simulink model "four_bit_adder"  (R2017a)
settings: Solver=VariableStepAuto  StartTime=0.0  StopTime=10.0  RelTol=1e-3
settings Model: Creator=nailt  LastModifiedBy=nailt

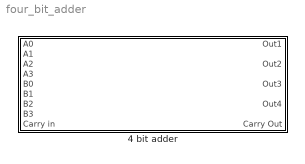
== system four_bit_adder ==
  4 bit adder : Subsystem

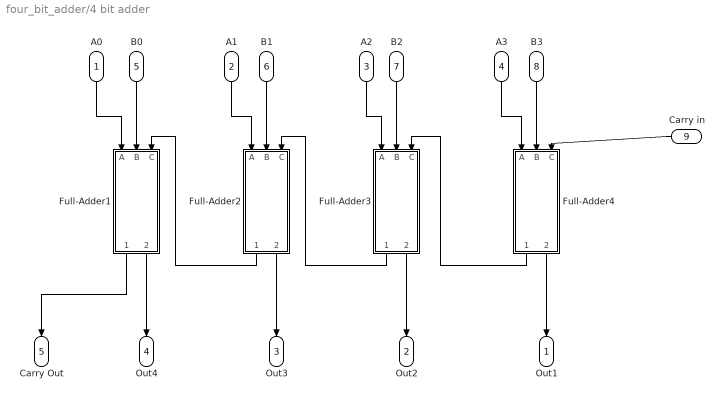
== system four_bit_adder/4 bit adder ==
  "A0 " : Inport
  "A1 " : Inport  Port=2
  A2 : Inport  Port=3
  A3 : Inport  Port=4
  B0 : Inport  Port=5
  B1 : Inport  Port=6
  B2 : Inport  Port=7
  B3 : Inport  Port=8
  Carry in : Inport  Port=9
  Full-Adder1 : Subsystem
  Full-Adder2 : Subsystem
  Full-Adder3 : Subsystem
  Full-Adder4 : Subsystem
  Out1 : Outport
  Out2 : Outport  Port=2
  Out3 : Outport  Port=3
  Out4 : Outport  Port=4
  Carry Out : Outport  Port=5
  wires:
  B3/1 -> Full-Adder4/2(B)
  B2/1 -> Full-Adder3/2(B)
  Full-Adder1/1(CARRY) -> Carry Out/1
  A3/1 -> Full-Adder4/1(A)
  "A1 "/1 -> Full-Adder2/1(A)
  Full-Adder2/1(CARRY) -> Full-Adder1/3(C)
  "A0 "/1 -> Full-Adder1/1(A)
  Full-Adder3/2(OUTPUT) -> Out2/1
  B1/1 -> Full-Adder2/2(B)
  Full-Adder4/2(OUTPUT) -> Out1/1
  Full-Adder2/2(OUTPUT) -> Out3/1
  Carry in/1 -> Full-Adder4/3(C)
  Full-Adder1/2(OUTPUT) -> Out4/1
  Full-Adder4/1(CARRY) -> Full-Adder3/3(C)
  A2/1 -> Full-Adder3/1(A)
  Full-Adder3/1(CARRY) -> Full-Adder2/3(C)
  B0/1 -> Full-Adder1/2(B)

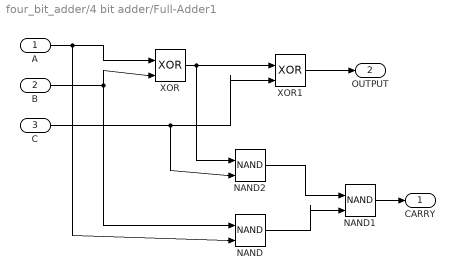
== system four_bit_adder/4 bit adder/Full-Adder1 ==
  A : Inport
  B : Inport  Port=2
  C : Inport  Port=3
  NAND : Logic  Operator=NAND  IconShape=distinctive  AllPortsSameDT=off  OutDataTypeStr=boolean
  NAND1 : Logic  Operator=NAND  IconShape=distinctive  AllPortsSameDT=off  OutDataTypeStr=boolean
  NAND2 : Logic  Operator=NAND  IconShape=distinctive  AllPortsSameDT=off  OutDataTypeStr=boolean
  XOR : Logic  Operator=XOR  IconShape=distinctive  AllPortsSameDT=off  OutDataTypeStr=boolean
  XOR1 : Logic  Operator=XOR  IconShape=distinctive  AllPortsSameDT=off  OutDataTypeStr=boolean
  CARRY : Outport
  OUTPUT : Outport  Port=2
  wires:
  C/1 -> NAND2/2, XOR1/2
  XOR1/1 -> OUTPUT/1
  A/1 -> NAND/2, XOR/1
  B/1 -> NAND/1, XOR/2
  NAND/1 -> NAND1/2
  NAND1/1 -> CARRY/1
  NAND2/1 -> NAND1/1
  XOR/1 -> NAND2/1, XOR1/1

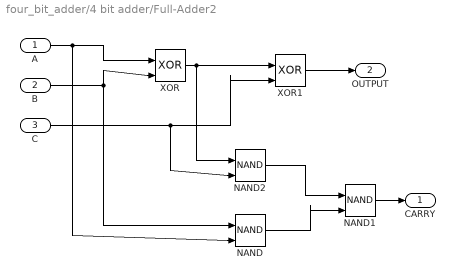
== system four_bit_adder/4 bit adder/Full-Adder2 ==
  A : Inport
  B : Inport  Port=2
  C : Inport  Port=3
  NAND : Logic  Operator=NAND  IconShape=distinctive  AllPortsSameDT=off  OutDataTypeStr=boolean
  NAND1 : Logic  Operator=NAND  IconShape=distinctive  AllPortsSameDT=off  OutDataTypeStr=boolean
  NAND2 : Logic  Operator=NAND  IconShape=distinctive  AllPortsSameDT=off  OutDataTypeStr=boolean
  XOR : Logic  Operator=XOR  IconShape=distinctive  AllPortsSameDT=off  OutDataTypeStr=boolean
  XOR1 : Logic  Operator=XOR  IconShape=distinctive  AllPortsSameDT=off  OutDataTypeStr=boolean
  CARRY : Outport
  OUTPUT : Outport  Port=2
  wires:
  C/1 -> NAND2/2, XOR1/2
  XOR1/1 -> OUTPUT/1
  A/1 -> NAND/2, XOR/1
  B/1 -> NAND/1, XOR/2
  NAND/1 -> NAND1/2
  NAND1/1 -> CARRY/1
  NAND2/1 -> NAND1/1
  XOR/1 -> NAND2/1, XOR1/1

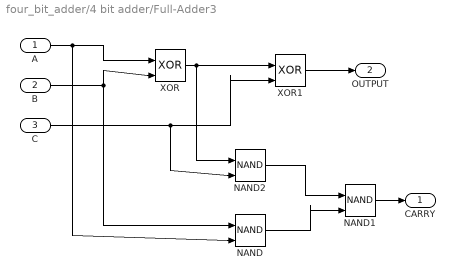
== system four_bit_adder/4 bit adder/Full-Adder3 ==
  A : Inport
  B : Inport  Port=2
  C : Inport  Port=3
  NAND : Logic  Operator=NAND  IconShape=distinctive  AllPortsSameDT=off  OutDataTypeStr=boolean
  NAND1 : Logic  Operator=NAND  IconShape=distinctive  AllPortsSameDT=off  OutDataTypeStr=boolean
  NAND2 : Logic  Operator=NAND  IconShape=distinctive  AllPortsSameDT=off  OutDataTypeStr=boolean
  XOR : Logic  Operator=XOR  IconShape=distinctive  AllPortsSameDT=off  OutDataTypeStr=boolean
  XOR1 : Logic  Operator=XOR  IconShape=distinctive  AllPortsSameDT=off  OutDataTypeStr=boolean
  CARRY : Outport
  OUTPUT : Outport  Port=2
  wires:
  C/1 -> NAND2/2, XOR1/2
  XOR1/1 -> OUTPUT/1
  A/1 -> NAND/2, XOR/1
  B/1 -> NAND/1, XOR/2
  NAND/1 -> NAND1/2
  NAND1/1 -> CARRY/1
  NAND2/1 -> NAND1/1
  XOR/1 -> NAND2/1, XOR1/1

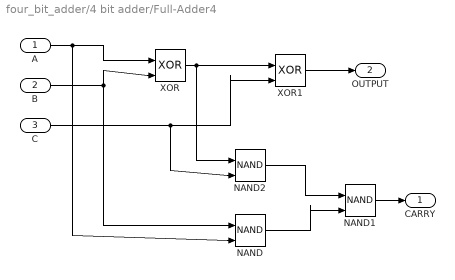
== system four_bit_adder/4 bit adder/Full-Adder4 ==
  A : Inport
  B : Inport  Port=2
  C : Inport  Port=3
  NAND : Logic  Operator=NAND  IconShape=distinctive  AllPortsSameDT=off  OutDataTypeStr=boolean
  NAND1 : Logic  Operator=NAND  IconShape=distinctive  AllPortsSameDT=off  OutDataTypeStr=boolean
  NAND2 : Logic  Operator=NAND  IconShape=distinctive  AllPortsSameDT=off  OutDataTypeStr=boolean
  XOR : Logic  Operator=XOR  IconShape=distinctive  AllPortsSameDT=off  OutDataTypeStr=boolean
  XOR1 : Logic  Operator=XOR  IconShape=distinctive  AllPortsSameDT=off  OutDataTypeStr=boolean
  CARRY : Outport
  OUTPUT : Outport  Port=2
  wires:
  C/1 -> NAND2/2, XOR1/2
  XOR1/1 -> OUTPUT/1
  A/1 -> NAND/2, XOR/1
  B/1 -> NAND/1, XOR/2
  NAND/1 -> NAND1/2
  NAND1/1 -> CARRY/1
  NAND2/1 -> NAND1/1
  XOR/1 -> NAND2/1, XOR1/1
